simulink model "beam_control_ic_rx"  (R2022b)
settings: Solver=VariableStepAuto  StartTime=0.0  StopTime=136e-9  RelTol=1e-3
values from neighbouring files (symbols this model uses):
  Bias = 0    [ModelingRFSystemsWithAntennaArraysUsingAntennaBlockExample.m]    (also in beam_control_ic_rx_parameter.m)
  filter_gain0_0 = 0    [ModelingRFSystemsWithAntennaArraysUsingAntennaBlockExample.m]    (also in beam_control_ic_rx_parameter.m)
  filter_gain0_1 = 1/6    (= 0.166666666667)    [ModelingRFSystemsWithAntennaArraysUsingAntennaBlockExample.m]    (also in beam_control_ic_rx_parameter.m)
  filter_gain0_2 = 2/3    (= 0.666666666667)    [ModelingRFSystemsWithAntennaArraysUsingAntennaBlockExample.m]    (also in beam_control_ic_rx_parameter.m)
  filter_gain0_3 = 1/6    (= 0.166666666667)    [ModelingRFSystemsWithAntennaArraysUsingAntennaBlockExample.m]    (also in beam_control_ic_rx_parameter.m)
  filter_gain1_0 = 0    [ModelingRFSystemsWithAntennaArraysUsingAntennaBlockExample.m]    (also in beam_control_ic_rx_parameter.m)
  filter_gain1_1 = 1/2    (= 0.5)    [ModelingRFSystemsWithAntennaArraysUsingAntennaBlockExample.m]    (also in beam_control_ic_rx_parameter.m)
  filter_gain1_2 = 0    [ModelingRFSystemsWithAntennaArraysUsingAntennaBlockExample.m]    (also in beam_control_ic_rx_parameter.m)
  filter_gain1_3 = -1/2    (= -0.5)    [ModelingRFSystemsWithAntennaArraysUsingAntennaBlockExample.m]    (also in beam_control_ic_rx_parameter.m)
  filter_gain2_0 = 0    [ModelingRFSystemsWithAntennaArraysUsingAntennaBlockExample.m]    (also in beam_control_ic_rx_parameter.m)
  filter_gain2_1 = 1/2    (= 0.5)    [ModelingRFSystemsWithAntennaArraysUsingAntennaBlockExample.m]    (also in beam_control_ic_rx_parameter.m)
  filter_gain2_2 = -1    [ModelingRFSystemsWithAntennaArraysUsingAntennaBlockExample.m]    (also in beam_control_ic_rx_parameter.m)
  filter_gain2_3 = 1/2    (= 0.5)    [ModelingRFSystemsWithAntennaArraysUsingAntennaBlockExample.m]    (also in beam_control_ic_rx_parameter.m)
  filter_gain3_0 = 1/6    (= 0.166666666667)    [ModelingRFSystemsWithAntennaArraysUsingAntennaBlockExample.m]    (also in beam_control_ic_rx_parameter.m)
  filter_gain3_1 = -1/2    (= -0.5)    [ModelingRFSystemsWithAntennaArraysUsingAntennaBlockExample.m]    (also in beam_control_ic_rx_parameter.m)
  filter_gain3_2 = 1/2    (= 0.5)    [ModelingRFSystemsWithAntennaArraysUsingAntennaBlockExample.m]    (also in beam_control_ic_rx_parameter.m)
  filter_gain3_3 = -1/6    (= -0.166666666667)    [ModelingRFSystemsWithAntennaArraysUsingAntennaBlockExample.m]    (also in beam_control_ic_rx_parameter.m)
  fraction_delay = 1.5    [ModelingRFSystemsWithAntennaArraysUsingAntennaBlockExample.m]    (also in beam_control_ic_rx_parameter.m = 1)
  integer_delay = 0    [ModelingRFSystemsWithAntennaArraysUsingAntennaBlockExample.m]    (also in beam_control_ic_rx_parameter.m)
  N = 10    [ModelingRFSystemsWithAntennaArraysUsingAntennaBlockExample.m]    (also in beam_control_ic_rx_parameter.m)
  Ref = 2.048    [ModelingRFSystemsWithAntennaArraysUsingAntennaBlockExample.m]    (also in beam_control_ic_rx_parameter.m)
  rx_amplitude_compensation = 1    [ModelingRFSystemsWithAntennaArraysUsingAntennaBlockExample.m]    (also in beam_control_ic_rx_parameter.m)
  rx_freq_d_compensation = 250e6    (= 250000000)    [ModelingRFSystemsWithAntennaArraysUsingAntennaBlockExample.m]    (also in beam_control_ic_rx_parameter.m)
  rx_phase_compensation = 0    [ModelingRFSystemsWithAntennaArraysUsingAntennaBlockExample.m]    (also in beam_control_ic_rx_parameter.m)
undefined symbols (not defined in the file or in its folder): fdesignblkfcn, gcbh, pskmod
libraries: dspsigops x5, simulink_extras x3, dspmlti4 x3, msbDacArchitectures x2, commrfcorlib x1, commeq3 x1
(part 3 of 3)

== system beam_control_ic_rx/Digital_Compensation3/TTD_Farrow1/Cubic Lagrange Interpolator3 ==
  In1 : Inport
  Delay6 : Delay  DelayLength=1
  Delay7 : Delay  DelayLength=1
  Delay8 : Delay  DelayLength=1
  Gain : Gain  Gain=filter_gain3_3
  Gain1 : Gain  Gain=filter_gain3_2
  Gain2 : Gain  Gain=filter_gain3_1
  Gain3 : Gain  Gain=filter_gain3_0
  Sum : Sum  Inputs=++|
  Sum2 : Sum  Inputs=++|
  Sum3 : Sum  Inputs=++|
  Out1 : Outport
  wires:
  Sum3/1 -> Out1/1
  Gain3/1 -> Sum3/1
  Sum/1 -> Sum2/2
  Gain/1 -> Sum/2
  Delay8/1 -> Gain3/1
  In1/1 -> Delay6/1, Gain/1
  Gain2/1 -> Sum2/1
  Sum2/1 -> Sum3/2
  Delay7/1 -> Gain2/1, Delay8/1
  Delay6/1 -> Gain1/1, Delay7/1
  Gain1/1 -> Sum/1
